simulink model "model1input"  (R2019a)
settings: Solver=VariableStepAuto  StartTime=0.0  StopTime=5  RelTol=1e-3
values from neighbouring files (symbols this model uses):
  A = [-c/ms c/ms;c/mu -c/mu]    [Part12b.m]    (also in Part33DofPar.m = [a11 a12 a13 a14; Part3BicyclePar.m = [-(caf+car)/(u*M) -((a*caf-b*car)/(u*M)+u); part23.m = [a11 a12 a13)
  B = [-ks/ms ks/ms;ks/mu -ks/mu-kt/mu]    [Part12b.m]    (also in Part33DofPar.m = [b1;b2;b3;b4]; Part3BicyclePar.m = [caf/M;a*caf/Iz]; part23.m = [b1;b2;b4])
  c = 800    [Part12b.m]
  C = [0;kt/mu]    [Part12b.m]
  kf = 12861    [Part12b.m]
  mf = 269.231    [Part12b.m]

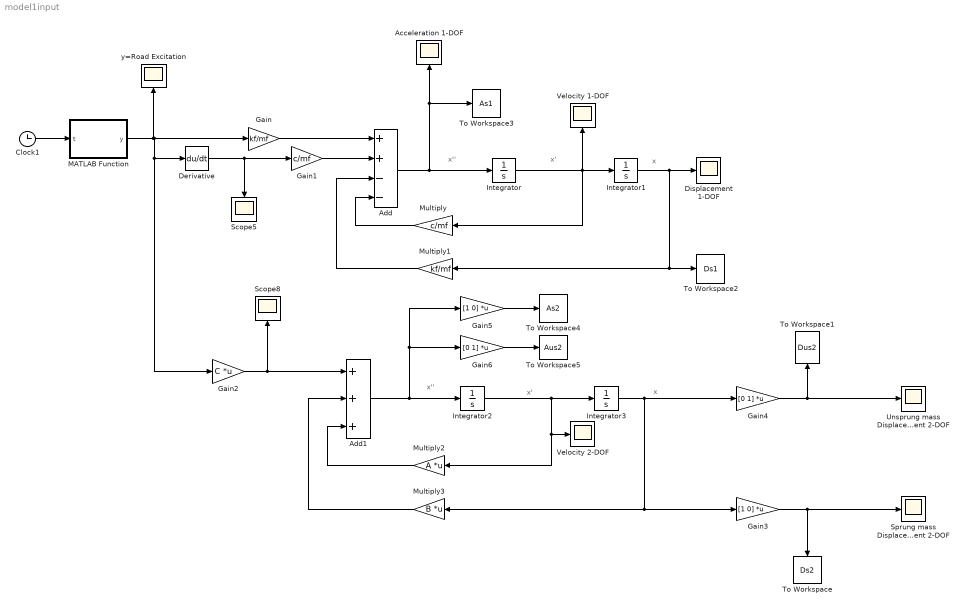
== system model1input ==
  note: x
  note: x'
  note: x''
  note: x
  note: x'
  note: x''
  " y=Road Excitation" : Scope
  Acceleration 1-DOF : Scope
  Add : Sum  Inputs=++--
  Add1 : Sum  Inputs=+++
  Clock1 : Clock
  Derivative : Derivative
  Displacement 1-DOF : Scope
  Gain : Gain  Gain=kf/mf
  Gain1 : Gain  Gain=c/mf
  Gain2 : Gain  Gain=C  Multiplication=Matrix(K*u)
  Gain3 : Gain  Gain=[1 0]  Multiplication=Matrix(K*u)
  Gain4 : Gain  Gain=[0 1]  Multiplication=Matrix(K*u)
  Gain5 : Gain  Gain=[1 0]  Multiplication=Matrix(K*u)
  Gain6 : Gain  Gain=[0 1]  Multiplication=Matrix(K*u)
  Integrator{,1..3} (4 alike) : Integrator
  MATLAB Function : MATLAB Function  TreatAsAtomicUnit=on
  Multiply : Gain  Gain=c/mf
  Multiply1 : Gain  Gain=kf/mf
  Multiply2 : Gain  Gain=A  Multiplication=Matrix(K*u)
  Multiply3 : Gain  Gain=B  Multiplication=Matrix(K*u)
  Scope5 : Scope
  Scope8 : Scope
  Sprung mass Displacement 2-DOF : Scope
  To Workspace : ToWorkspace  VariableName=Ds2  SaveFormat=Timeseries  SampleTime=-1
  To Workspace1 : ToWorkspace  VariableName=Dus2  SaveFormat=Timeseries  SampleTime=-1
  To Workspace2 : ToWorkspace  VariableName=Ds1  SaveFormat=Timeseries  SampleTime=-1
  To Workspace3 : ToWorkspace  VariableName=As1  SaveFormat=Timeseries  SampleTime=-1
  To Workspace4 : ToWorkspace  VariableName=As2  SaveFormat=Timeseries  SampleTime=-1
  To Workspace5 : ToWorkspace  VariableName=Aus2  SaveFormat=Timeseries  SampleTime=-1
  Unsprung mass Displacement 2-DOF : Scope
  Velocity 1-DOF : Scope
  Velocity 2-DOF : Scope
  wires:
  Add/1 -> Integrator/1, Acceleration 1-DOF/1, To Workspace3/1
  Integrator/1 -> Multiply/1, Velocity 1-DOF/1, Integrator1/1
  Integrator1/1 -> Displacement 1-DOF/1, To Workspace2/1, Multiply1/1
  Clock1/1 -> MATLAB Function/1(t)
  MATLAB Function/1(y) -> Gain/1, Gain2/1, Derivative/1, " y=Road Excitation"/1
  Gain/1 -> Add/1
  Gain2/1 -> Add1/1, Scope8/1
  Add1/1 -> Gain6/1, Gain5/1, Integrator2/1
  Integrator2/1 -> Multiply2/1, Velocity 2-DOF/1, Integrator3/1
  Integrator3/1 -> Multiply3/1, Gain3/1, Gain4/1
  Derivative/1 -> Gain1/1, Scope5/1
  Multiply2/1 -> Add1/3
  Multiply3/1 -> Add1/2
  Gain1/1 -> Add/2
  Multiply/1 -> Add/4
  Multiply1/1 -> Add/3
  Gain3/1 -> To Workspace/1, Sprung mass Displacement 2-DOF/1
  Gain4/1 -> To Workspace1/1, Unsprung mass Displacement 2-DOF/1
  Gain5/1 -> To Workspace4/1
  Gain6/1 -> To Workspace5/1

== matlab function model1input/MATLAB Function ==
  data: t input; y output
function y = fcn(t)
x=50/3.6*t;

if x<0.6
    y=0.1*sin(pi*(x)/0.6);
    %y=0.1*0.5*(1-cos(2*pi*x/1.2));
else
    y=0;
end
